simulink model "Analysis"  (R2024b)
settings: Solver=ode45  StartTime=0.0  StopTime=5  RelTol=1e-3
values from neighbouring files (symbols this model uses):
  B = 0    [Constants.m]
  J = 1    [Constants.m]
  K = 1    [Constants.m]
  L = 12*(10^(-3))    (= 0.012)    [Constants.m]
  R = 240    [Constants.m]
  V = 240    [Constants.m]
settings Model: Creator=ThinkPad  LastModifiedBy=ThinkPad

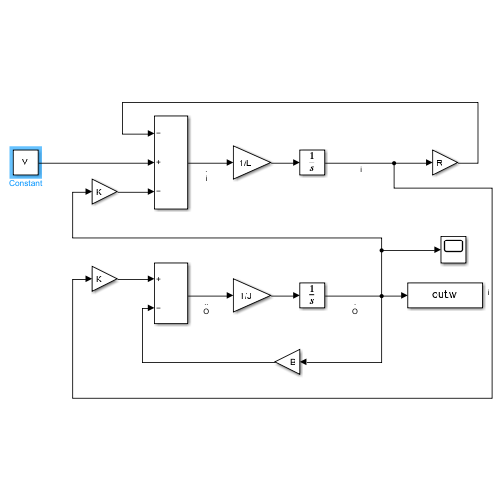
[thumbnail: Simulink's stored preview of the top-level diagram]
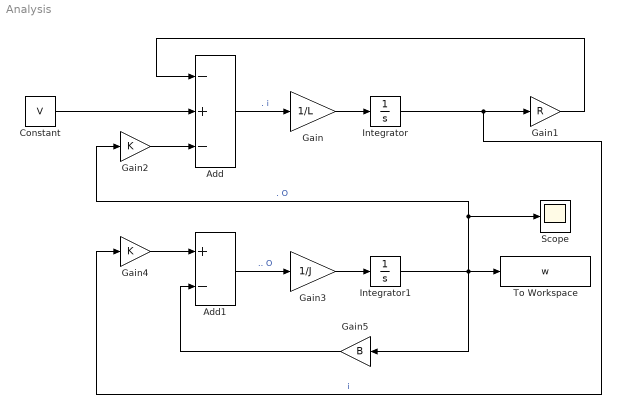
== system Analysis ==
  Add : Sum  Inputs=-+-
  Add1 : Sum  Inputs=+-
  Constant : Constant  Value=V
  Gain : Gain  Gain=1/L
  Gain1 : Gain  Gain=R
  Gain2 : Gain  Gain=K
  Gain3 : Gain  Gain=1/J
  Gain4 : Gain  Gain=K
  Gain5 : Gain  Gain=B
  Integrator : Integrator
  Integrator1 : Integrator
  Scope : Scope
  To Workspace : ToWorkspace  VariableName=w  SaveFormat=Structure With Time  SampleTime=-1
  wires:
  Gain/1 -> Integrator/1
  Add/1 -> Gain/1  ". i"
  Integrator/1 -> Gain1/1, Gain4/1  "i"
  Gain3/1 -> Integrator1/1
  Add1/1 -> Gain3/1  ".. O"
  Integrator1/1 -> To Workspace/1, Scope/1, Gain2/1, Gain5/1  ". O"
  Gain5/1 -> Add1/2
  Constant/1 -> Add/2
  Gain1/1 -> Add/1
  Gain2/1 -> Add/3
  Gain4/1 -> Add1/1
